simulink model "Speed_Controller_Test_gr2"  (Simulink 7.0)
settings: Solver=ode4  SolverMode=SingleTasking  StartTime=0.0  StopTime=252  FixedStep=0.01  RelTol=1e-3
InitFcn:
  | tempomat_para
StopFcn:
  | clear;
values from neighbouring files (symbols this model uses):
  A = 1.9    [tempomat_para.m]
  a_Fzg_max = 2    [tempomat_para.m]
  a_Fzg_min = -2    [tempomat_para.m]
  cw = 0.32    [tempomat_para.m]
  gang = [1 2 3 4]    [tempomat_para.m]
  gang_vec = [1 2 3 4]    [tempomat_para.m]
  i_anteil = 5    [tempomat_para.m]
  i_d = 3.42    [tempomat_para.m]
  i_g = [3.91 2.17 1.37 1.00]    [tempomat_para.m]
  lambda_gang = [1.3 1.25  1.17  1.05]    [tempomat_para.m]
  m_Fzg = 1400    [tempomat_para.m]
  M_mot_max = [130 149 163 170 168 166 162 158 150 139 123 80]    [tempomat_para.m]
  M_mot_min = [0 -40]    [tempomat_para.m]
  n_mot0 = 1000    [tempomat_para.m]
  n_mot_max = 1000:500:6500    [tempomat_para.m]
  n_mot_min = [1000 6500]    [tempomat_para.m]
  p_anteil = 100    [tempomat_para.m]
  r_dyn = 0.28    [tempomat_para.m]
  rho = 1.202    [tempomat_para.m]
  t_sch = 0.2    [tempomat_para.m]
  TI = [block '/TI']    [PSTI_callback.m]
  v_Fzg_ms0 = 0    [tempomat_para.m]
undefined symbols (not defined in the file or in its folder): Drossel_mat, getdatatypespecs
libraries: simulink x116, fzgbib x3
(part 6 of 10)

== system Speed_Controller_Test_gr2/Test Specification/R2 Speed Control velocity restoration time after simple  acceleration/deceleration/after (6 seconds)  |V_Des-V_Vhcl <= 1.4|/PAS2/Ra delay ==
  In1 : Inport  OutDataType=sfix(16)  OutScaling=2^0
  Data Type Conversion : DataTypeConversion  OutDataType=sfix(16)  OutScaling=2^0
  Delay : Constant  Value=0  OutDataType=sfix(16)  OutScaling=2^0
  Integer Delay : S-Function  FunctionName=sfix_udelay  Parameters=samptime,vinit,NumDelays,1,1,0  mask(Integer Delay){vinit=0.0, samptime=-1, NumDelays=15}
      mask prompts: vinit "Initial condition:"; samptime "Sample time:"; NumDelays "Number of delays:"
      mask help: Delay a signal N sample periods.
      mask init:
      | if isempty(NumDelays)
      |    NumDelays = 1;
      | end
      mask Display: fprintf(' %d\nZ   ',-1*(NumDelays))
  Switch : Switch  Criteria=u2 ~= 0
  Out1 : Outport  OutDataType=sfix(16)  OutScaling=2^0
  wires:
  Switch/1 -> Data Type Conversion/1
  In1/1 -> Switch/3, Integer Delay/1
  Delay/1 -> Switch/2
  Integer Delay/1 -> Switch/1
  Data Type Conversion/1 -> Out1/1

== system Speed_Controller_Test_gr2/Test Specification/R2 Speed Control velocity restoration time after simple  acceleration/deceleration/after (6 seconds)  |V_Des-V_Vhcl <= 1.4|/PAS2/Rp delay ==
  In1 : Inport  OutDataType=sfix(16)  OutScaling=2^0
  Data Type Conversion : DataTypeConversion  OutDataType=sfix(16)  OutScaling=2^0
  Delay : Constant  Value=600  OutDataType=sfix(16)  OutScaling=2^0
  Integer Delay : S-Function  FunctionName=sfix_udelay  Parameters=samptime,vinit,NumDelays,1,1,0  mask(Integer Delay){vinit=0.0, samptime=-1, NumDelays=600}
      mask prompts: vinit "Initial condition:"; samptime "Sample time:"; NumDelays "Number of delays:"
      mask help: Delay a signal N sample periods.
      mask init:
      | if isempty(NumDelays)
      |    NumDelays = 1;
      | end
      mask Display: fprintf(' %d\nZ   ',-1*(NumDelays))
  Switch : Switch  Criteria=u2 ~= 0
  Out1 : Outport  OutDataType=sfix(16)  OutScaling=2^0
  wires:
  Switch/1 -> Data Type Conversion/1
  In1/1 -> Switch/3, Integer Delay/1
  Delay/1 -> Switch/2
  Integer Delay/1 -> Switch/1
  Data Type Conversion/1 -> Out1/1

== system Speed_Controller_Test_gr2/Test Specification/R2 Speed Control velocity restoration time after simple  acceleration/deceleration/after (6 seconds)  |V_Des-V_Vhcl <= 1.4|/PAS2/Ta delay ==
  In1 : Inport  OutDataType=sfix(16)  OutScaling=2^0
  Data Type Conversion : DataTypeConversion  OutDataType=sfix(16)  OutScaling=2^0
  Delay : Constant  Value=0  OutDataType=sfix(16)  OutScaling=2^0
  Integer Delay : S-Function  FunctionName=sfix_udelay  Parameters=samptime,vinit,NumDelays,1,1,0  mask(Integer Delay){vinit=0.0, samptime=-1, NumDelays=15}
      mask prompts: vinit "Initial condition:"; samptime "Sample time:"; NumDelays "Number of delays:"
      mask help: Delay a signal N sample periods.
      mask init:
      | if isempty(NumDelays)
      |    NumDelays = 1;
      | end
      mask Display: fprintf(' %d\nZ   ',-1*(NumDelays))
  Switch : Switch  Criteria=u2 ~= 0
  Out1 : Outport  OutDataType=sfix(16)  OutScaling=2^0
  wires:
  Switch/1 -> Data Type Conversion/1
  In1/1 -> Switch/3, Integer Delay/1
  Delay/1 -> Switch/2
  Integer Delay/1 -> Switch/1
  Data Type Conversion/1 -> Out1/1

== system Speed_Controller_Test_gr2/Test Specification/R2 Speed Control velocity restoration time after simple  acceleration/deceleration/after (6 seconds)  |V_Des-V_Vhcl <= 1.4|/PAS2/Tp delay ==
  In1 : Inport  OutDataType=sfix(16)  OutScaling=2^0
  Data Type Conversion : DataTypeConversion  OutDataType=sfix(16)  OutScaling=2^0
  Delay : Constant  Value=600  OutDataType=sfix(16)  OutScaling=2^0
  Integer Delay : S-Function  FunctionName=sfix_udelay  Parameters=samptime,vinit,NumDelays,1,1,0  mask(Integer Delay){vinit=0.0, samptime=-1, NumDelays=600}
      mask prompts: vinit "Initial condition:"; samptime "Sample time:"; NumDelays "Number of delays:"
      mask help: Delay a signal N sample periods.
      mask init:
      | if isempty(NumDelays)
      |    NumDelays = 1;
      | end
      mask Display: fprintf(' %d\nZ   ',-1*(NumDelays))
  Switch : Switch  Criteria=u2 ~= 0
  Out1 : Outport  OutDataType=sfix(16)  OutScaling=2^0
  wires:
  Switch/1 -> Data Type Conversion/1
  In1/1 -> Switch/3, Integer Delay/1
  Delay/1 -> Switch/2
  Integer Delay/1 -> Switch/1
  Data Type Conversion/1 -> Out1/1

== system Speed_Controller_Test_gr2/Test Specification/R2 Speed Control velocity restoration time after simple  acceleration/deceleration/after (6 seconds)  |V_Des-V_Vhcl <= 1.4|/PAS2/V delay ==
  In1 : Inport  OutDataType=sfix(16)  OutScaling=2^0
  Data Type Conversion : DataTypeConversion  OutDataType=sfix(16)  OutScaling=2^0
  Delay : Constant  Value=0  OutDataType=sfix(16)  OutScaling=2^0
  Integer Delay : S-Function  FunctionName=sfix_udelay  Parameters=samptime,vinit,NumDelays,1,1,0  mask(Integer Delay){vinit=0.0, samptime=-1, NumDelays=15}
      mask prompts: vinit "Initial condition:"; samptime "Sample time:"; NumDelays "Number of delays:"
      mask help: Delay a signal N sample periods.
      mask init:
      | if isempty(NumDelays)
      |    NumDelays = 1;
      | end
      mask Display: fprintf(' %d\nZ   ',-1*(NumDelays))
  Switch : Switch  Criteria=u2 ~= 0
  Out1 : Outport  OutDataType=sfix(16)  OutScaling=2^0
  wires:
  Switch/1 -> Data Type Conversion/1
  In1/1 -> Switch/3, Integer Delay/1
  Delay/1 -> Switch/2
  Integer Delay/1 -> Switch/1
  Data Type Conversion/1 -> Out1/1

== system Speed_Controller_Test_gr2/Test Specification/R2 Speed Control velocity restoration time after simple  acceleration/deceleration/after (6 seconds)  |V_Des-V_Vhcl <= 1.4|/PAS2/error ==
  Rp : Inport  OutDataType=sfix(16)  OutScaling=2^0
  Tp : Inport  Port=2  OutDataType=sfix(16)  OutScaling=2^0
  A : Inport  Port=3  OutDataType=sfix(16)  OutScaling=2^0
  Ra : Inport  Port=4  OutDataType=sfix(16)  OutScaling=2^0
  Ta : Inport  Port=5  OutDataType=sfix(16)  OutScaling=2^0
  V : Inport  Port=6  OutDataType=sfix(16)  OutScaling=2^0
  Compare To Constant{,2,4,6,8,10} (6 alike) : simulink/Logic and Bit Operations/Compare To Constant  SystemSampleTime=-1  relop===  const=0  LogicOutDataTypeMode=uint8  ZeroCross=off
  Compare To Constant{1,3,5,7,9,11} (6 alike) : simulink/Logic and Bit Operations/Compare To Constant  SystemSampleTime=-1  relop===  const=1  LogicOutDataTypeMode=uint8  ZeroCross=off
  Logical Operator{,1,3..6} (6 alike) : Logic  Operator=NOR  AllPortsSameDT=off  OutDataTypeMode=boolean
  Logical Operator2 : Logic  Operator=OR  Inputs=6  AllPortsSameDT=off  OutDataTypeMode=boolean
  Verror : Outport  OutDataType=sfix(16)  OutScaling=2^0
  wires:
  Compare To Constant9/1 -> Logical Operator5/2
  Compare To Constant8/1 -> Logical Operator5/1
  Ta/1 -> Compare To Constant8/1, Compare To Constant9/1
  Compare To Constant7/1 -> Logical Operator4/2
  Compare To Constant6/1 -> Logical Operator4/1
  Ra/1 -> Compare To Constant7/1, Compare To Constant6/1
  Tp/1 -> Compare To Constant3/1, Compare To Constant2/1
  Rp/1 -> Compare To Constant1/1, Compare To Constant/1
  Logical Operator2/1 -> Verror/1
  Compare To Constant3/1 -> Logical Operator1/2
  Compare To Constant2/1 -> Logical Operator1/1
  Compare To Constant1/1 -> Logical Operator/2
  Compare To Constant/1 -> Logical Operator/1
  Compare To Constant5/1 -> Logical Operator3/2
  Compare To Constant4/1 -> Logical Operator3/1
  A/1 -> Compare To Constant4/1, Compare To Constant5/1
  Compare To Constant11/1 -> Logical Operator6/2
  Compare To Constant10/1 -> Logical Operator6/1
  V/1 -> Compare To Constant10/1, Compare To Constant11/1
  Logical Operator/1 -> Logical Operator2/1
  Logical Operator1/1 -> Logical Operator2/2
  Logical Operator3/1 -> Logical Operator2/3
  Logical Operator4/1 -> Logical Operator2/4
  Logical Operator5/1 -> Logical Operator2/5
  Logical Operator6/1 -> Logical Operator2/6

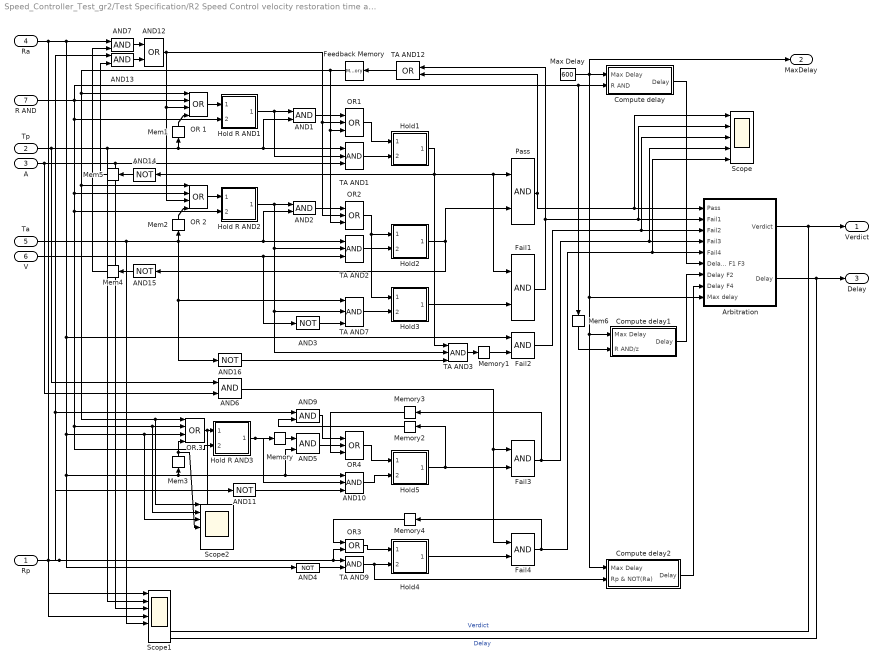
== system Speed_Controller_Test_gr2/Test Specification/R2 Speed Control velocity restoration time after simple  acceleration/deceleration/after (6 seconds)  |V_Des-V_Vhcl <= 1.4|/PAS2/none - pass - fail ==
  Rp : Inport  OutDataType=sfix(16)  OutScaling=2^0
  Tp : Inport  Port=2  OutDataType=sfix(16)  OutScaling=2^0
  A : Inport  Port=3  OutDataType=sfix(16)  OutScaling=2^0
  Ra : Inport  Port=4  OutDataType=sfix(16)  OutScaling=2^0
  Ta : Inport  Port=5  OutDataType=sfix(16)  OutScaling=2^0
  V : Inport  Port=6  OutDataType=sfix(16)  OutScaling=2^0
  R AND : Inport  Port=7  OutDataType=sfix(16)  OutScaling=2^0
  AND{1..2,5..7,9,13} (7 alike) : Logic  AllPortsSameDT=off  OutDataTypeMode=boolean
  AND10 : Logic  Inputs=3  AllPortsSameDT=off  OutDataTypeMode=boolean
  AND{3..4,11,16} (4 alike) : Logic  Operator=NOT  AllPortsSameDT=off  OutDataTypeMode=boolean
  AND12 : Logic  Operator=OR  AllPortsSameDT=off  OutDataTypeMode=boolean
  AND14 : Logic  Orientation=left  Operator=NOT  AllPortsSameDT=off  OutDataTypeMode=boolean
  AND15 : Logic  Orientation=left  Operator=NOT  AllPortsSameDT=off  OutDataTypeMode=boolean
  Arbitration : Subsystem
  Compute delay : Subsystem
  Compute delay1 : Subsystem
  Compute delay2 : Subsystem
  Fail{1..4} (4 alike) : Logic  AllPortsSameDT=off  OutDataTypeMode=boolean
  Feedback Memory : Memory  Orientation=left
  Hold R AND1 : Subsystem  TreatAsAtomicUnit=on
      mask Display: patch(-0.31+[0.4 0.46 0.46 0.54 0.54 0.6 0.6 0.55 0.55 0.45 0.45 0.4],-0.19+[0.85 0.85 0.95 0.95 0.85 0.85 0.87 0.87 0.96 0.96 0.87 0.87],[0 0 0]);
  Hold R AND2 : Subsystem  TreatAsAtomicUnit=on
      mask Display: patch(-0.31+[0.4 0.46 0.46 0.54 0.54 0.6 0.6 0.55 0.55 0.45 0.45 0.4],-0.19+[0.85 0.85 0.95 0.95 0.85 0.85 0.87 0.87 0.96 0.96 0.87 0.87],[0 0 0]);
  Hold R AND3 : Subsystem  TreatAsAtomicUnit=on
      mask Display: patch(-0.31+[0.4 0.46 0.46 0.54 0.54 0.6 0.6 0.55 0.55 0.45 0.45 0.4],-0.19+[0.85 0.85 0.95 0.95 0.85 0.85 0.87 0.87 0.96 0.96 0.87 0.87],[0 0 0]);
  Hold1 : Subsystem  TreatAsAtomicUnit=on
      mask Display: patch(-0.31+[0.4 0.46 0.46 0.54 0.54 0.6 0.6 0.55 0.55 0.45 0.45 0.4],-0.19+[0.85 0.85 0.95 0.95 0.85 0.85 0.87 0.87 0.96 0.96 0.87 0.87],[0 0 0]);
  Hold2 : Subsystem  TreatAsAtomicUnit=on
      mask Display: patch(-0.31+[0.4 0.46 0.46 0.54 0.54 0.6 0.6 0.55 0.55 0.45 0.45 0.4],-0.19+[0.85 0.85 0.95 0.95 0.85 0.85 0.87 0.87 0.96 0.96 0.87 0.87],[0 0 0]);
  Hold3 : Subsystem  TreatAsAtomicUnit=on
      mask Display: patch(-0.31+[0.4 0.46 0.46 0.54 0.54 0.6 0.6 0.55 0.55 0.45 0.45 0.4],-0.19+[0.85 0.85 0.95 0.95 0.85 0.85 0.87 0.87 0.96 0.96 0.87 0.87],[0 0 0]);
  Hold4 : Subsystem  TreatAsAtomicUnit=on
      mask Display: patch(-0.31+[0.4 0.46 0.46 0.54 0.54 0.6 0.6 0.55 0.55 0.45 0.45 0.4],-0.19+[0.85 0.85 0.95 0.95 0.85 0.85 0.87 0.87 0.96 0.96 0.87 0.87],[0 0 0]);
  Hold5 : Subsystem  TreatAsAtomicUnit=on
      mask Display: patch(-0.31+[0.4 0.46 0.46 0.54 0.54 0.6 0.6 0.55 0.55 0.45 0.45 0.4],-0.19+[0.85 0.85 0.95 0.95 0.85 0.85 0.87 0.87 0.96 0.96 0.87 0.87],[0 0 0]);
  Max Delay : Constant  Value=600  OutDataType=sfix(16)  OutScaling=2^0
  Mem1 : Memory  Orientation=up
  Mem2 : Memory  Orientation=up
  Mem3 : Memory  Orientation=up
  Mem4 : Memory  Orientation=left
  Mem5 : Memory  Orientation=left
  Mem6 : Memory  Orientation=down
  Memory : Memory
  Memory1 : Memory
  Memory2 : Memory  Orientation=left
  Memory3 : Memory  Orientation=left
  Memory4 : Memory  Orientation=left
  OR 1 : Logic  Operator=OR  Inputs=4  AllPortsSameDT=off  OutDataTypeMode=boolean
  OR 2 : Logic  Operator=OR  Inputs=4  AllPortsSameDT=off  OutDataTypeMode=boolean
  OR 3 : Logic  Operator=OR  Inputs=4  AllPortsSameDT=off  OutDataTypeMode=boolean
  OR1 : Logic  Operator=OR  Inputs=3  AllPortsSameDT=off  OutDataTypeMode=boolean
  OR2 : Logic  Operator=OR  Inputs=3  AllPortsSameDT=off  OutDataTypeMode=boolean
  OR3 : Logic  Operator=OR  AllPortsSameDT=off  OutDataTypeMode=boolean
  OR4 : Logic  Operator=OR  Inputs=3  AllPortsSameDT=off  OutDataTypeMode=boolean
  Pass : Logic  AllPortsSameDT=off  OutDataTypeMode=boolean
  Scope : Scope  NumInputPorts=5
      settings: YMin=-5~-5~-5~-5~-5  YMax=5~5~5~5~5  SaveName=ScopeData9  MaxDataPoints=1115000
  Scope1 : Scope  NumInputPorts=7
      settings: YMin=-5~-5~-5~-5~-5~-5~-5  YMax=5~5~5~5~5~5~5  SaveName=ScopeData10  MaxDataPoints=1115000
  Scope2 : Scope  NumInputPorts=7
      settings: YMin=-5~-5~-5~-5~-5~-5~-5  YMax=5~5~5~5~5~5~5  SaveName=ScopeData11  MaxDataPoints=1115000
  TA AND{1..3,7} (4 alike) : Logic  Inputs=3  AllPortsSameDT=off  OutDataTypeMode=boolean
  TA AND12 : Logic  Orientation=left  Operator=OR  AllPortsSameDT=off  OutDataTypeMode=boolean
  TA AND9 : Logic  AllPortsSameDT=off  OutDataTypeMode=boolean
  Verdict : Outport  OutDataType=sfix(16)  OutScaling=2^0
  MaxDelay : Outport  Port=2  OutDataType=sfix(16)  OutScaling=2^0
  Delay : Outport  Port=3  OutDataType=sfix(16)  OutScaling=2^0
  wires:
  Arbitration/2(Delay) -> Delay/1, Scope1/7  "Delay"
  Arbitration/1(Verdict) -> Verdict/1, Scope1/6  "Verdict"
  Compute delay2/1(Delay) -> Arbitration/8(Delay F4)
  Compute delay1/1(Delay) -> Arbitration/7(Delay F2)
  Compute delay/1(Delay) -> Arbitration/6(Delay P F1 F3)
  Mem6/1 -> Compute delay1/2(R AND/z)
  AND6/1 -> Fail4/1, Fail3/1
  Max Delay/1 -> MaxDelay/1, Compute delay/1(Max Delay), Arbitration/9(Max delay), Compute delay1/1(Max Delay), Compute delay2/1(Max Delay)
  Memory4/1 -> OR3/1
  OR3/1 -> Hold4/1(" ")
  Pass/1 -> TA AND12/2, Arbitration/1(Pass), Scope/1
  AND16/1 -> TA AND3/3
  Fail1/1 -> TA AND12/1, Arbitration/2(Fail1), Scope/2
  AND15/1 -> Mem4/1
  AND14/1 -> Mem5/1
  Mem5/1 -> AND13/2
  Mem4/1 -> AND7/2
  AND12/1 -> OR2/2, OR1/2, OR 2/3, OR 1/3
  AND13/1 -> AND12/2
  AND7/1 -> AND12/1
  AND5/1 -> OR4/2
  AND10/1 -> Hold5/2("    ")
  AND11/1 -> AND10/3
  Memory3/1 -> OR4/3
  Memory2/1 -> AND9/2
  AND9/1 -> OR4/1
  Memory1/1 -> Fail2/2
  Fail2/1 -> Arbitration/3(Fail2), Scope/3
  Fail4/1 -> Memory4/1, Arbitration/5(Fail4), Scope/5
  Fail3/1 -> Memory3/1, Arbitration/4(Fail3), Scope/4
  TA AND12/1 -> Feedback Memory/1
  Hold5/1("  ") -> Fail3/2, Memory2/1
  Mem3/1 -> OR 3/4, Scope2/4
  OR 3/1 -> Hold R AND3/1(" "), Scope2/5
  Hold R AND3/1("  ") -> Memory/1, AND10/2
  OR4/1 -> Hold5/1(" ")
  Hold4/1("  ") -> Fail4/2
  TA AND9/1 -> Compute delay2/2(Rp & NOT(Ra)), Hold4/2("    ")
  Rp/1 -> OR3/2, TA AND9/1, AND13/1, AND11/1, AND9/1, Scope1/1
  AND4/1 -> TA AND9/2
  Hold3/1("  ") -> Fail1/2
  TA AND3/1 -> Memory1/1
  AND3/1 -> TA AND7/3
  TA AND7/1 -> Hold3/2("    ")
  Mem2/1 -> OR 2/4
  Mem1/1 -> OR 1/4
  Ra/1 -> AND7/1, AND4/1, Mem3/1, AND5/2, AND10/1, OR 3/3, Scope2/3, Fail2/1, Scope1/4
  R AND/1 -> Mem6/1, Compute delay/2(R AND), OR 1/2, Hold R AND1/2("    "), Hold R AND3/2("    "), OR 3/2, Scope2/2, Hold R AND2/2("    "), OR 2/2
  Feedback Memory/1 -> OR2/3, OR1/3, OR 2/1, OR 3/1, Scope2/1, OR 1/1
  AND2/1 -> OR2/1
  Hold R AND2/1("  ") -> TA AND2/2, TA AND7/2, TA AND3/2, AND2/1
  TA AND2/1 -> Hold2/2("    ")
  OR2/1 -> Hold3/1(" "), Hold2/1(" ")
  Hold2/1("  ") -> Pass/2, AND15/1
  V/1 -> TA AND2/3, AND3/1
  OR 2/1 -> Hold R AND2/1(" ")
  Ta/1 -> TA AND2/1, AND2/2, AND16/1, TA AND7/1, Mem2/1, Scope1/5
  AND1/1 -> OR1/1
  Hold R AND1/1("  ") -> TA AND1/2, AND1/1
  TA AND1/1 -> Hold1/2("    ")
  OR1/1 -> Hold1/1(" ")
  Hold1/1("  ") -> TA AND3/1, AND14/1, Fail1/1, Pass/1
  A/1 -> AND6/2, TA AND1/3, Scope1/3
  OR 1/1 -> Hold R AND1/1(" ")
  Tp/1 -> AND6/1, AND1/2, TA AND1/1, Mem1/1, Scope1/2
  Memory/1 -> AND5/1

== system Speed_Controller_Test_gr2/Test Specification/R2 Speed Control velocity restoration time after simple  acceleration/deceleration/after (6 seconds)  |V_Des-V_Vhcl <= 1.4|/R = 2/Active for  6s after R=1  ==
  Signal 2 : Inport  OutDataType=sfix(16)  OutScaling=2^0
  Memory : Memory
  Min Time : Constant  Value=6  OutDataType=sfix(16)  OutScaling=2^0
  Relational Operator2 : RelationalOperator  LogicOutDataTypeMode=boolean
  Scope : Scope  NumInputPorts=5
      settings: YMin=-1~154~-5~80~0  YMax=1~163~5~107.5~110  SaveName=ScopeData13  MaxDataPoints=5000000
  Switch : Switch  Threshold=1
  Time since R = 1 : Subsystem  TreatAsAtomicUnit=on
  Zero : Constant  Value=0  OutDataType=sfix(16)  OutScaling=2^0
  6s after : Outport  OutDataType=sfix(16)  OutScaling=2^0
  wires:
  Relational Operator2/1 -> 6s after/1, Scope/4
  Min Time/1 -> Relational Operator2/1
  Switch/1 -> Relational Operator2/2, Scope/3
  Time since R = 1/1(Trigger) -> Scope/1, Switch/2
  Zero/1 -> Switch/3
  Signal 2/1 -> Time since R = 1/1(Signal)
  Time since R = 1/2(Feature) -> Memory/1
  Memory/1 -> Switch/1, Scope/2

== system Speed_Controller_Test_gr2/Test Specification/R2 Speed Control velocity restoration time after simple  acceleration/deceleration/after (6 seconds)  |V_Des-V_Vhcl <= 1.4|/R = 2/Hold1 ==
  " " : Inport  OutDataType=sfix(16)  OutScaling=2^0
  "    " : Inport  Port=2  OutDataType=sfix(16)  OutScaling=2^0
  Constant : Constant  Value=0  OutDataType=sfix(16)  OutScaling=2^0
  Switch : Switch  Criteria=u2 ~= 0
  "  " : Outport  OutDataType=sfix(16)  OutScaling=2^0
  wires:
  Switch/1 -> "  "/1
  "    "/1 -> Switch/1
  " "/1 -> Switch/2
  Constant/1 -> Switch/3

== system Speed_Controller_Test_gr2/Test Specification/R2 Speed Control velocity restoration time after simple  acceleration/deceleration/after (6 seconds)  |V_Des-V_Vhcl <= 1.4|/R = 2/Hold2 ==
  " " : Inport  OutDataType=sfix(16)  OutScaling=2^0
  "    " : Inport  Port=2  OutDataType=sfix(16)  OutScaling=2^0
  Constant : Constant  Value=0  OutDataType=sfix(16)  OutScaling=2^0
  Switch : Switch  Criteria=u2 ~= 0
  "  " : Outport  OutDataType=sfix(16)  OutScaling=2^0
  wires:
  Switch/1 -> "  "/1
  "    "/1 -> Switch/1
  " "/1 -> Switch/2
  Constant/1 -> Switch/3

== system Speed_Controller_Test_gr2/Test Specification/R2 Speed Control velocity restoration time after simple  acceleration/deceleration/after (6 seconds)  |V_Des-V_Vhcl <= 1.4|/R = 2/R = 1 ==
  In1 : Inport  OutDataType=sfix(16)  OutScaling=2^0
  Bus Selector1 : BusSelector  OutputSignals=R
  Constant : Constant  OutDataType=sfix(16)  OutScaling=2^0
  Relational Operator : RelationalOperator  Operator===  LogicOutDataTypeMode=boolean
  Out1 : Outport  OutDataType=sfix(16)  OutScaling=2^0
  wires:
  In1/1 -> Bus Selector1/1
  Constant/1 -> Relational Operator/2
  Bus Selector1/1 -> Relational Operator/1  "<R>"
  Relational Operator/1 -> Out1/1

== system Speed_Controller_Test_gr2/Test Specification/R1 Speed Control step response/Complete step & CC active + no target & Speed Control active/Complete step detection/Step detection/Active if signals constant for some specified time ==
  Signal1 : Inport  OutDataType=sfix(16)  OutScaling=2^0
  Signal 2 : Inport  Port=2  OutDataType=sfix(16)  OutScaling=2^0
  Logical Operator1 : Logic  AllPortsSameDT=off  OutDataTypeMode=boolean
  Min Time : Constant  Value=10  OutDataType=sfix(16)  OutScaling=2^0
  MinMax : MinMax  Inputs=2  OutDataType=sfix(16)  OutScaling=2^0
  Relational Operator2 : RelationalOperator  Operator=<=  LogicOutDataTypeMode=boolean
  Switch : Switch  Criteria=u2 ~= 0
  Time since signal constant : Subsystem  TreatAsAtomicUnit=on  mask(Feature extraction block){RT=0.001}
      mask prompts: RT "Relative tolerance in %"
      mask help: Detect if the signal value is constant (using the last two signal values) allowing for a user-defined relative deviation
      mask CallbackString:
      | if or( (str2double(get_param(gcb,'RT')) < 0), (str2double(get_param(gcb,'RT')) > 100))
      |     error(['Relative tolerance value (' get_param(gcb,'RT') ') out of range. Please give a value between 0 and 100.']);
      | else
      |     set_param([gcb '/Detect constant/Relative tolerance/Relative Tolerance'],'Value',get_param(gcb,'RT'));
      |     set_param([gcb '/Detect constant'],'RT',get_param(gcb,'RT'));
      | end
  Time since signal constant1 : Subsystem  TreatAsAtomicUnit=on  mask(Feature extraction block){RT=0.001}
      mask prompts: RT "Relative tolerance in %"
      mask help: Detect if the signal value is constant (using the last two signal values) allowing for a user-defined relative deviation
      mask CallbackString:
      | if or( (str2double(get_param(gcb,'RT')) < 0), (str2double(get_param(gcb,'RT')) > 100))
      |     error(['Relative tolerance value (' get_param(gcb,'RT') ') out of range. Please give a value between 0 and 100.']);
      | else
      |     set_param([gcb '/Detect constant/Relative tolerance/Relative Tolerance'],'Value',get_param(gcb,'RT'));
      |     set_param([gcb '/Detect constant'],'RT',get_param(gcb,'RT'));
      | end
  Zero : Constant  Value=0  OutDataType=sfix(16)  OutScaling=2^0
  Constant signals : Outport  OutDataType=sfix(16)  OutScaling=2^0
  wires:
  Zero/1 -> Switch/3
  Logical Operator1/1 -> Switch/2
  MinMax/1 -> Switch/1
  Time since signal constant1/1(Trigger) -> Logical Operator1/2
  Time since signal constant/1(Trigger) -> Logical Operator1/1
  Time since signal constant/2(Feature) -> MinMax/1
  Time since signal constant1/2(Feature) -> MinMax/2
  Switch/1 -> Relational Operator2/2
  Min Time/1 -> Relational Operator2/1
  Relational Operator2/1 -> Constant signals/1
  Signal 2/1 -> Time since signal constant1/1(Signal)
  Signal1/1 -> Time since signal constant/1(Signal)

== system Speed_Controller_Test_gr2/Test Specification/R1 Speed Control step response/Complete step & CC active + no target & Speed Control active/Complete step detection/Step detection/Detect constant ==
  Signal : Inport  OutDataType=sfix(16)  OutScaling=2^0
  Clock : Clock
      settings: Decimation=10
  Constant1 : Constant  Value=0  OutDataTypeMode=boolean  OutDataType=sfix(16)  OutScaling=2^0
  Memory : Memory
  Relative tolerance : Subsystem
  Switch : Switch  Criteria=u2 > Threshold
  Constant : Outport  OutDataType=sfix(16)  OutScaling=2^0
  wires:
  Signal/1 -> Memory/1, Relative tolerance/1(sig)
  Memory/1 -> Relative tolerance/2(ref)
  Constant1/1 -> Switch/3
  Clock/1 -> Switch/2
  Relative tolerance/1(sig == ref) -> Switch/1
  Switch/1 -> Constant/1

== system Speed_Controller_Test_gr2/Test Specification/R1 Speed Control step response/Complete step & CC active + no target & Speed Control active/Complete step detection/Step detection/Detect decrease ==
  Signal : Inport  OutDataType=sfix(16)  OutScaling=2^0
  Clock : Clock
      settings: Decimation=10
  Memory : Memory
  Relational Operator : RelationalOperator  Operator=<  LogicOutDataTypeMode=Specify via dialog
  Switch : Switch  Criteria=u2 > Threshold
  Decrease : Outport  OutDataType=sfix(16)  OutScaling=2^0
  wires:
  Signal/1 -> Relational Operator/1, Memory/1, Switch/3
  Relational Operator/1 -> Decrease/1
  Clock/1 -> Switch/2
  Memory/1 -> Switch/1
  Switch/1 -> Relational Operator/2

== system Speed_Controller_Test_gr2/Test Specification/R1 Speed Control step response/Complete step & CC active + no target & Speed Control active/Complete step detection/Step detection/Detect increase ==
  Signal : Inport  OutDataType=sfix(16)  OutScaling=2^0
  Clock : Clock
      settings: Decimation=10
  Memory : Memory
  Relational Operator : RelationalOperator  Operator=>  LogicOutDataTypeMode=Specify via dialog
  Switch : Switch  Criteria=u2 > Threshold
  Increase : Outport  OutDataType=sfix(16)  OutScaling=2^0
  wires:
  Switch/1 -> Relational Operator/2
  Memory/1 -> Switch/1
  Clock/1 -> Switch/2
  Relational Operator/1 -> Increase/1
  Signal/1 -> Switch/3, Memory/1, Relational Operator/1

== system Speed_Controller_Test_gr2/Test Specification/R1 Speed Control step response/Complete step & CC active + no target & Speed Control active/Complete step detection/Step detection/Detect increase2 ==
  Signal : Inport  OutDataType=sfix(16)  OutScaling=2^0
  Clock : Clock
      settings: Decimation=10
  Memory : Memory
  Relational Operator : RelationalOperator  Operator=>  LogicOutDataTypeMode=Specify via dialog
  Switch : Switch  Criteria=u2 > Threshold
  Increase : Outport  OutDataType=sfix(16)  OutScaling=2^0
  wires:
  Signal/1 -> Relational Operator/1, Memory/1, Switch/3
  Relational Operator/1 -> Increase/1
  Clock/1 -> Switch/2
  Memory/1 -> Switch/1
  Switch/1 -> Relational Operator/2

== system Speed_Controller_Test_gr2/Test Specification/R1 Speed Control step response/Complete step & CC active + no target & Speed Control active/Complete step detection/Step detection/Hold1 ==
  " " : Inport  OutDataType=sfix(16)  OutScaling=2^0
  "    " : Inport  Port=2  OutDataType=sfix(16)  OutScaling=2^0
  Memory : Memory  Orientation=left
  Switch : Switch  Criteria=u2 ~= 0
  "  " : Outport  OutDataType=sfix(16)  OutScaling=2^0
  wires:
  " "/1 -> Switch/2
  "    "/1 -> Switch/1
  Switch/1 -> "  "/1, Memory/1
  Memory/1 -> Switch/3

== system Speed_Controller_Test_gr2/Test Specification/R1 Speed Control step response/Complete step & CC active + no target & Speed Control active/Complete step detection/Step detection reset/Active if signals constant for some specified time ==
  Signal1 : Inport  OutDataType=sfix(16)  OutScaling=2^0
  Signal 2 : Inport  Port=2  OutDataType=sfix(16)  OutScaling=2^0
  Logical Operator1 : Logic  AllPortsSameDT=off  OutDataTypeMode=boolean
  Min Time : Constant  Value=10  OutDataType=sfix(16)  OutScaling=2^0
  MinMax : MinMax  Inputs=2  OutDataType=sfix(16)  OutScaling=2^0
  Relational Operator2 : RelationalOperator  Operator=<=  LogicOutDataTypeMode=boolean
  Switch : Switch  Criteria=u2 ~= 0
  Time since signal constant : Subsystem  TreatAsAtomicUnit=on  mask(Feature extraction block){RT=0.0001}
      mask prompts: RT "Relative tolerance in %"
      mask help: Detect if the signal value is constant (using the last two signal values) allowing for a user-defined relative deviation
      mask CallbackString:
      | if or( (str2double(get_param(gcb,'RT')) < 0), (str2double(get_param(gcb,'RT')) > 100))
      |     error(['Relative tolerance value (' get_param(gcb,'RT') ') out of range. Please give a value between 0 and 100.']);
      | else
      |     set_param([gcb '/Detect constant/Relative tolerance/Relative Tolerance'],'Value',get_param(gcb,'RT'));
      |     set_param([gcb '/Detect constant'],'RT',get_param(gcb,'RT'));
      | end
  Time since signal constant1 : Subsystem  TreatAsAtomicUnit=on  mask(Feature extraction block){RT=0.0001}
      mask prompts: RT "Relative tolerance in %"
      mask help: Detect if the signal value is constant (using the last two signal values) allowing for a user-defined relative deviation
      mask CallbackString:
      | if or( (str2double(get_param(gcb,'RT')) < 0), (str2double(get_param(gcb,'RT')) > 100))
      |     error(['Relative tolerance value (' get_param(gcb,'RT') ') out of range. Please give a value between 0 and 100.']);
      | else
      |     set_param([gcb '/Detect constant/Relative tolerance/Relative Tolerance'],'Value',get_param(gcb,'RT'));
      |     set_param([gcb '/Detect constant'],'RT',get_param(gcb,'RT'));
      | end
  Zero : Constant  Value=0  OutDataType=sfix(16)  OutScaling=2^0
  Constant signals : Outport  OutDataType=sfix(16)  OutScaling=2^0
  wires:
  Signal1/1 -> Time since signal constant/1(Signal)
  Signal 2/1 -> Time since signal constant1/1(Signal)
  Relational Operator2/1 -> Constant signals/1
  Min Time/1 -> Relational Operator2/1
  Switch/1 -> Relational Operator2/2
  Time since signal constant1/2(Feature) -> MinMax/2
  Time since signal constant/2(Feature) -> MinMax/1
  Time since signal constant/1(Trigger) -> Logical Operator1/1
  Time since signal constant1/1(Trigger) -> Logical Operator1/2
  MinMax/1 -> Switch/1
  Logical Operator1/1 -> Switch/2
  Zero/1 -> Switch/3

== system Speed_Controller_Test_gr2/Test Specification/R1 Speed Control step response/Complete step & CC active + no target & Speed Control active/Complete step detection/Step detection reset/Step detection ==
  Signal : Inport  OutDataType=sfix(16)  OutScaling=2^0
  Abs : Abs
  Add : Sum  Inputs=+-  OutDataType=sfix(16)  OutScaling=2^-10
  Clock : Clock
      settings: Decimation=10
  Memory : Memory
  Min step size : Constant  Value=10  OutDataType=sfix(16)  OutScaling=2^0
  Relational Operator : RelationalOperator  LogicOutDataTypeMode=boolean
  Switch : Switch  Criteria=u2 > Threshold
  Step : Outport  OutDataType=sfix(16)  OutScaling=2^0
  wires:
  Add/1 -> Abs/1
  Relational Operator/1 -> Step/1
  Min step size/1 -> Relational Operator/2
  Abs/1 -> Relational Operator/1
  Signal/1 -> Memory/1, Switch/3, Add/1
  Clock/1 -> Switch/2
  Memory/1 -> Switch/1
  Switch/1 -> Add/2

== system Speed_Controller_Test_gr2/Test Specification/R1 Speed Control step response/Complete step & CC active + no target & Speed Control active/PS/TI/Delays1 ==
  In1 : Inport  OutDataType=sfix(16)  OutScaling=2^0
  Delay : Constant  Value=0  OutDataType=sfix(16)  OutScaling=2^0
  Integer Delay : S-Function  FunctionName=sfix_udelay  Parameters=samptime,vinit,NumDelays,1,1,0  mask(Integer Delay){vinit=0.0, samptime=-1, NumDelays=15}
      mask prompts: vinit "Initial condition:"; samptime "Sample time:"; NumDelays "Number of delays:"
      mask help: Delay a signal N sample periods.
      mask init:
      | if isempty(NumDelays)
      |    NumDelays = 1;
      | end
      mask Display: fprintf(' %d\nZ   ',-1*(NumDelays))
  Switch : Switch  Criteria=u2 ~= 0
  Out1 : Outport  OutDataType=sfix(16)  OutScaling=2^0
  wires:
  Integer Delay/1 -> Switch/1
  Delay/1 -> Switch/2
  In1/1 -> Integer Delay/1, Switch/3
  Switch/1 -> Out1/1

== system Speed_Controller_Test_gr2/Test Specification/R1 Speed Control step response/Complete step & CC active + no target & Speed Control active/PS/TI/Delays2 ==
  In1 : Inport  OutDataType=sfix(16)  OutScaling=2^0
  Delay : Constant  Value=0  OutDataType=sfix(16)  OutScaling=2^0
  Integer Delay : S-Function  FunctionName=sfix_udelay  Parameters=samptime,vinit,NumDelays,1,1,0  mask(Integer Delay){vinit=0.0, samptime=-1, NumDelays=15}
      mask prompts: vinit "Initial condition:"; samptime "Sample time:"; NumDelays "Number of delays:"
      mask help: Delay a signal N sample periods.
      mask init:
      | if isempty(NumDelays)
      |    NumDelays = 1;
      | end
      mask Display: fprintf(' %d\nZ   ',-1*(NumDelays))
  Switch : Switch  Criteria=u2 ~= 0
  Out1 : Outport  OutDataType=sfix(16)  OutScaling=2^0
  wires:
  Integer Delay/1 -> Switch/1
  Delay/1 -> Switch/2
  In1/1 -> Integer Delay/1, Switch/3
  Switch/1 -> Out1/1

== system Speed_Controller_Test_gr2/Test Specification/R1 Speed Control step response/Complete step & CC active + no target & Speed Control active/PS/TID/Hold R AND1 ==
  " " : Inport  OutDataType=sfix(16)  OutScaling=2^0
  "    " : Inport  Port=2  OutDataType=sfix(16)  OutScaling=2^0
  Memory : Memory  Orientation=left
  Switch : Switch  Criteria=u2 ~= 0
  "  " : Outport  OutDataType=sfix(16)  OutScaling=2^0
  wires:
  Memory/1 -> Switch/3
  Switch/1 -> Memory/1, "  "/1
  "    "/1 -> Switch/1
  " "/1 -> Switch/2

== system Speed_Controller_Test_gr2/Test Specification/R1 Speed Control step response/Complete step & CC active + no target & Speed Control active/PS/TID/Hold1 ==
  " " : Inport  OutDataType=sfix(16)  OutScaling=2^0
  "    " : Inport  Port=2  OutDataType=sfix(16)  OutScaling=2^0
  Memory : Memory  Orientation=left
  Switch : Switch  Criteria=u2 ~= 0
  "  " : Outport  OutDataType=sfix(16)  OutScaling=2^0
  wires:
  Memory/1 -> Switch/3
  Switch/1 -> Memory/1, "  "/1
  "    "/1 -> Switch/1
  " "/1 -> Switch/2

== system Speed_Controller_Test_gr2/Test Specification/R1 Speed Control step response/Maximum overshoot < 5 &  Steady state error < 5/PAS/Delay bus signals/AD delay ==
  In1 : Inport  OutDataType=sfix(16)  OutScaling=2^0
  Delay : Constant  Value=0  OutDataType=sfix(16)  OutScaling=2^0
  Integer Delay : S-Function  FunctionName=sfix_udelay  Parameters=samptime,vinit,NumDelays,1,1,0  mask(Integer Delay){vinit=0.0, samptime=-1, NumDelays=15}
      mask prompts: vinit "Initial condition:"; samptime "Sample time:"; NumDelays "Number of delays:"
      mask help: Delay a signal N sample periods.
      mask init:
      | if isempty(NumDelays)
      |    NumDelays = 1;
      | end
      mask Display: fprintf(' %d\nZ   ',-1*(NumDelays))
  Switch : Switch  Criteria=u2 ~= 0
  Out1 : Outport  OutDataType=sfix(16)  OutScaling=2^0
  wires:
  Switch/1 -> Out1/1
  In1/1 -> Switch/3, Integer Delay/1
  Delay/1 -> Switch/2
  Integer Delay/1 -> Switch/1

== system Speed_Controller_Test_gr2/Test Specification/R1 Speed Control step response/Maximum overshoot < 5 &  Steady state error < 5/PAS/Delay bus signals/ELL delay ==
  In1 : Inport  OutDataType=sfix(16)  OutScaling=2^0
  Delay : Constant  Value=0  OutDataType=sfix(16)  OutScaling=2^0
  Integer Delay : S-Function  FunctionName=sfix_udelay  Parameters=samptime,vinit,NumDelays,1,1,0  mask(Integer Delay){vinit=0.0, samptime=-1, NumDelays=15}
      mask prompts: vinit "Initial condition:"; samptime "Sample time:"; NumDelays "Number of delays:"
      mask help: Delay a signal N sample periods.
      mask init:
      | if isempty(NumDelays)
      |    NumDelays = 1;
      | end
      mask Display: fprintf(' %d\nZ   ',-1*(NumDelays))
  Switch : Switch  Criteria=u2 ~= 0
  Out1 : Outport  OutDataType=sfix(16)  OutScaling=2^0
  wires:
  Switch/1 -> Out1/1
  In1/1 -> Switch/3, Integer Delay/1
  Delay/1 -> Switch/2
  Integer Delay/1 -> Switch/1

== system Speed_Controller_Test_gr2/Test Specification/R1 Speed Control step response/Maximum overshoot < 5 &  Steady state error < 5/PAS/Delay bus signals/EUL delay ==
  In1 : Inport  OutDataType=sfix(16)  OutScaling=2^0
  Delay : Constant  Value=0  OutDataType=sfix(16)  OutScaling=2^0
  Integer Delay : S-Function  FunctionName=sfix_udelay  Parameters=samptime,vinit,NumDelays,1,1,0  mask(Integer Delay){vinit=0.0, samptime=-1, NumDelays=15}
      mask prompts: vinit "Initial condition:"; samptime "Sample time:"; NumDelays "Number of delays:"
      mask help: Delay a signal N sample periods.
      mask init:
      | if isempty(NumDelays)
      |    NumDelays = 1;
      | end
      mask Display: fprintf(' %d\nZ   ',-1*(NumDelays))
  Switch : Switch  Criteria=u2 ~= 0
  Out1 : Outport  OutDataType=sfix(16)  OutScaling=2^0
  wires:
  Integer Delay/1 -> Switch/1
  Delay/1 -> Switch/2
  In1/1 -> Integer Delay/1, Switch/3
  Switch/1 -> Out1/1

== system Speed_Controller_Test_gr2/Test Specification/R1 Speed Control step response/Maximum overshoot < 5 &  Steady state error < 5/PAS/none - pass - fail/Arbitration ==
  Pass : Inport  OutDataType=sfix(16)  OutScaling=2^0
  Fail1 : Inport  Port=2  OutDataType=sfix(16)  OutScaling=2^0
  Fail2 : Inport  Port=3  OutDataType=sfix(16)  OutScaling=2^0
  Fail3 : Inport  Port=4  OutDataType=sfix(16)  OutScaling=2^0
  Fail4 : Inport  Port=5  OutDataType=sfix(16)  OutScaling=2^0
  Delay P F1 F3 : Inport  Port=6  OutDataType=sfix(16)  OutScaling=2^0
  Delay F2 : Inport  Port=7  OutDataType=sfix(16)  OutScaling=2^0
  Delay F4 : Inport  Port=8  OutDataType=sfix(16)  OutScaling=2^0
  Max delay : Inport  Port=9  OutDataType=sfix(16)  OutScaling=2^0
  Verdict identification : Subsystem
  Verdict selection : Subsystem
  Verdict : Outport  OutDataType=sfix(16)  OutScaling=2^0
  Delay : Outport  Port=2  OutDataType=sfix(16)  OutScaling=2^0
  wires:
  Verdict selection/2(Delay) -> Delay/1
  Verdict selection/1(Verdict) -> Verdict/1
  Max delay/1 -> Verdict selection/6(Max delay)
  Verdict identification/2(V2) -> Verdict selection/2(V2)
  Verdict identification/1(V1) -> Verdict selection/1(V1)
  Delay F4/1 -> Verdict selection/5(Delay F4)
  Delay F2/1 -> Verdict selection/4(Delay F2)
  Delay P F1 F3/1 -> Verdict selection/3(Delay P F1 F3)
  Fail4/1 -> Verdict identification/5(Fail4)
  Fail3/1 -> Verdict identification/4(Fail3)
  Fail2/1 -> Verdict identification/3(Fail2)
  Fail1/1 -> Verdict identification/2(Fail1)
  Pass/1 -> Verdict identification/1(Pass)

== system Speed_Controller_Test_gr2/Test Specification/R1 Speed Control step response/Maximum overshoot < 5 &  Steady state error < 5/PAS/none - pass - fail/Compute delay ==
  Max Delay : Inport  OutDataType=sfix(16)  OutScaling=2^0
  R AND : Inport  Port=2  OutDataType=sfix(16)  OutScaling=2^0
  Clock : Clock
      settings: Decimation=10
  Clock1 : Clock
      settings: Decimation=10
  Divide : Product  Inputs=/*  OutDataType=sfix(16)  OutScaling=2^-10
  Hold1 : Subsystem  TreatAsAtomicUnit=on
      mask Display: patch(-0.31+[0.4 0.46 0.46 0.54 0.54 0.6 0.6 0.55 0.55 0.45 0.45 0.4],-0.19+[0.85 0.85 0.95 0.95 0.85 0.85 0.87 0.87 0.96 0.96 0.87 0.87],[0 0 0]);
  SimStepSize : Constant  Value=0.01  OutDataType=sfix(16)  OutScaling=2^0
  Subtract : Sum  Inputs=-+  OutDataType=sfix(16)  OutScaling=2^-10
  Subtract1 : Sum  Inputs=+-  OutDataType=sfix(16)  OutScaling=2^-10
  Delay : Outport  OutDataType=sfix(16)  OutScaling=2^0
  wires:
  Divide/1 -> Delay/1
  Max Delay/1 -> Subtract/1
  SimStepSize/1 -> Divide/1
  Clock/1 -> Hold1/2("    ")
  Subtract/1 -> Subtract1/2
  Subtract1/1 -> Divide/2
  Clock1/1 -> Subtract1/1
  Hold1/1("  ") -> Subtract/2
  R AND/1 -> Hold1/1(" ")

== system Speed_Controller_Test_gr2/Test Specification/R1 Speed Control step response/Maximum overshoot < 5 &  Steady state error < 5/PAS/none - pass - fail/Compute delay1 ==
  Max Delay : Inport  OutDataType=sfix(16)  OutScaling=2^0
  R AND/z : Inport  Port=2  OutDataType=sfix(16)  OutScaling=2^0
  Add : Sum  OutDataType=sfix(16)  OutScaling=2^-10
  Clock : Clock
      settings: Decimation=10
  Clock1 : Clock
      settings: Decimation=10
  Divide : Product  Inputs=/*  OutDataType=sfix(16)  OutScaling=2^-10
  Hold1 : Subsystem  TreatAsAtomicUnit=on
      mask Display: patch(-0.31+[0.4 0.46 0.46 0.54 0.54 0.6 0.6 0.55 0.55 0.45 0.45 0.4],-0.19+[0.85 0.85 0.95 0.95 0.85 0.85 0.87 0.87 0.96 0.96 0.87 0.87],[0 0 0]);
  SimStepSize : Constant  Value=0.01  OutDataType=sfix(16)  OutScaling=2^0
  Subtract : Sum  Inputs=-+  OutDataType=sfix(16)  OutScaling=2^-10
  Subtract1 : Sum  Inputs=+-  OutDataType=sfix(16)  OutScaling=2^-10
  Unit : Constant  OutDataType=sfix(16)  OutScaling=2^0
  Delay : Outport  OutDataType=sfix(16)  OutScaling=2^0
  wires:
  Divide/1 -> Add/2
  Unit/1 -> Add/1
  Max Delay/1 -> Subtract/1
  SimStepSize/1 -> Divide/1
  Clock/1 -> Hold1/2("    ")
  Subtract/1 -> Subtract1/2
  Subtract1/1 -> Divide/2
  Clock1/1 -> Subtract1/1
  Hold1/1("  ") -> Subtract/2
  R AND/z/1 -> Hold1/1(" ")
  Add/1 -> Delay/1

== system Speed_Controller_Test_gr2/Test Specification/R1 Speed Control step response/Maximum overshoot < 5 &  Steady state error < 5/PAS/none - pass - fail/Compute delay2 ==
  Max Delay : Inport  OutDataType=sfix(16)  OutScaling=2^0
  Rp & NOT(Ra) : Inport  Port=2  OutDataType=sfix(16)  OutScaling=2^0
  Clock : Clock
      settings: Decimation=10
  Clock1 : Clock
      settings: Decimation=10
  Divide : Product  Inputs=/*  OutDataType=sfix(16)  OutScaling=2^-10
  Hold1 : Subsystem  TreatAsAtomicUnit=on
      mask Display: patch(-0.31+[0.4 0.46 0.46 0.54 0.54 0.6 0.6 0.55 0.55 0.45 0.45 0.4],-0.19+[0.85 0.85 0.95 0.95 0.85 0.85 0.87 0.87 0.96 0.96 0.87 0.87],[0 0 0]);
  SimStepSize : Constant  Value=0.01  OutDataType=sfix(16)  OutScaling=2^0
  Subtract : Sum  Inputs=-+  OutDataType=sfix(16)  OutScaling=2^-10
  Subtract1 : Sum  Inputs=+-  OutDataType=sfix(16)  OutScaling=2^-10
  Delay : Outport  OutDataType=sfix(16)  OutScaling=2^0
  wires:
  Divide/1 -> Delay/1
  Rp & NOT(Ra)/1 -> Hold1/1(" ")
  Hold1/1("  ") -> Subtract/2
  Clock1/1 -> Subtract1/1
  Subtract1/1 -> Divide/2
  Subtract/1 -> Subtract1/2
  Clock/1 -> Hold1/2("    ")
  SimStepSize/1 -> Divide/1
  Max Delay/1 -> Subtract/1

== system Speed_Controller_Test_gr2/Test Specification/R1 Speed Control step response/Maximum overshoot < 5 &  Steady state error < 5/PAS/none - pass - fail/Hold R AND1 ==
  " " : Inport  OutDataType=sfix(16)  OutScaling=2^0
  "    " : Inport  Port=2  OutDataType=sfix(16)  OutScaling=2^0
  Memory : Memory  Orientation=left
  Switch : Switch  Criteria=u2 ~= 0
  "  " : Outport  OutDataType=sfix(16)  OutScaling=2^0
  wires:
  Memory/1 -> Switch/3
  Switch/1 -> Memory/1, "  "/1
  "    "/1 -> Switch/1
  " "/1 -> Switch/2

== system Speed_Controller_Test_gr2/Test Specification/R1 Speed Control step response/Maximum overshoot < 5 &  Steady state error < 5/PAS/none - pass - fail/Hold R AND2 ==
  " " : Inport  OutDataType=sfix(16)  OutScaling=2^0
  "    " : Inport  Port=2  OutDataType=sfix(16)  OutScaling=2^0
  Memory : Memory  Orientation=left
  Switch : Switch  Criteria=u2 ~= 0
  "  " : Outport  OutDataType=sfix(16)  OutScaling=2^0
  wires:
  Memory/1 -> Switch/3
  Switch/1 -> Memory/1, "  "/1
  "    "/1 -> Switch/1
  " "/1 -> Switch/2

== system Speed_Controller_Test_gr2/Test Specification/R1 Speed Control step response/Maximum overshoot < 5 &  Steady state error < 5/PAS/none - pass - fail/Hold R AND3 ==
  " " : Inport  OutDataType=sfix(16)  OutScaling=2^0
  "    " : Inport  Port=2  OutDataType=sfix(16)  OutScaling=2^0
  Memory : Memory  Orientation=left
  Switch : Switch  Criteria=u2 ~= 0
  "  " : Outport  OutDataType=sfix(16)  OutScaling=2^0
  wires:
  " "/1 -> Switch/2
  "    "/1 -> Switch/1
  Switch/1 -> "  "/1, Memory/1
  Memory/1 -> Switch/3

== system Speed_Controller_Test_gr2/Test Specification/R1 Speed Control step response/Maximum overshoot < 5 &  Steady state error < 5/PAS/none - pass - fail/Hold1 ==
  " " : Inport  OutDataType=sfix(16)  OutScaling=2^0
  "    " : Inport  Port=2  OutDataType=sfix(16)  OutScaling=2^0
  Memory : Memory  Orientation=left
  Switch : Switch  Criteria=u2 ~= 0
  "  " : Outport  OutDataType=sfix(16)  OutScaling=2^0
  wires:
  Memory/1 -> Switch/3
  Switch/1 -> Memory/1, "  "/1
  "    "/1 -> Switch/1
  " "/1 -> Switch/2

== system Speed_Controller_Test_gr2/Test Specification/R1 Speed Control step response/Maximum overshoot < 5 &  Steady state error < 5/PAS/none - pass - fail/Hold2 ==
  " " : Inport  OutDataType=sfix(16)  OutScaling=2^0
  "    " : Inport  Port=2  OutDataType=sfix(16)  OutScaling=2^0
  Memory : Memory  Orientation=left
  Switch : Switch  Criteria=u2 ~= 0
  "  " : Outport  OutDataType=sfix(16)  OutScaling=2^0
  wires:
  Memory/1 -> Switch/3
  Switch/1 -> Memory/1, "  "/1
  "    "/1 -> Switch/1
  " "/1 -> Switch/2

== system Speed_Controller_Test_gr2/Test Specification/R1 Speed Control step response/Maximum overshoot < 5 &  Steady state error < 5/PAS/none - pass - fail/Hold3 ==
  " " : Inport  OutDataType=sfix(16)  OutScaling=2^0
  "    " : Inport  Port=2  OutDataType=sfix(16)  OutScaling=2^0
  Memory : Memory  Orientation=left
  Switch : Switch  Criteria=u2 ~= 0
  "  " : Outport  OutDataType=sfix(16)  OutScaling=2^0
  wires:
  " "/1 -> Switch/2
  "    "/1 -> Switch/1
  Switch/1 -> "  "/1, Memory/1
  Memory/1 -> Switch/3

== system Speed_Controller_Test_gr2/Test Specification/R1 Speed Control step response/Maximum overshoot < 5 &  Steady state error < 5/PAS/none - pass - fail/Hold4 ==
  " " : Inport  OutDataType=sfix(16)  OutScaling=2^0
  "    " : Inport  Port=2  OutDataType=sfix(16)  OutScaling=2^0
  Memory : Memory  Orientation=left
  Switch : Switch  Criteria=u2 ~= 0
  "  " : Outport  OutDataType=sfix(16)  OutScaling=2^0
  wires:
  Memory/1 -> Switch/3
  Switch/1 -> Memory/1, "  "/1
  "    "/1 -> Switch/1
  " "/1 -> Switch/2

== system Speed_Controller_Test_gr2/Test Specification/R1 Speed Control step response/Maximum overshoot < 5 &  Steady state error < 5/PAS/none - pass - fail/Hold5 ==
  " " : Inport  OutDataType=sfix(16)  OutScaling=2^0
  "    " : Inport  Port=2  OutDataType=sfix(16)  OutScaling=2^0
  Memory : Memory  Orientation=left
  Switch : Switch  Criteria=u2 ~= 0
  "  " : Outport  OutDataType=sfix(16)  OutScaling=2^0
  wires:
  " "/1 -> Switch/2
  "    "/1 -> Switch/1
  Switch/1 -> "  "/1, Memory/1
  Memory/1 -> Switch/3

== system Speed_Controller_Test_gr2/Test Specification/R1 Speed Control step response/Maximum overshoot < 5 &  Steady state error < 5/PAS1/Delay bus signals/AD delay ==
  In1 : Inport  OutDataType=sfix(16)  OutScaling=2^0
  Delay : Constant  Value=0  OutDataType=sfix(16)  OutScaling=2^0
  Integer Delay : S-Function  FunctionName=sfix_udelay  Parameters=samptime,vinit,NumDelays,1,1,0  mask(Integer Delay){vinit=0.0, samptime=-1, NumDelays=15}
      mask prompts: vinit "Initial condition:"; samptime "Sample time:"; NumDelays "Number of delays:"
      mask help: Delay a signal N sample periods.
      mask init:
      | if isempty(NumDelays)
      |    NumDelays = 1;
      | end
      mask Display: fprintf(' %d\nZ   ',-1*(NumDelays))
  Switch : Switch  Criteria=u2 ~= 0
  Out1 : Outport  OutDataType=sfix(16)  OutScaling=2^0
  wires:
  Integer Delay/1 -> Switch/1
  Delay/1 -> Switch/2
  In1/1 -> Integer Delay/1, Switch/3
  Switch/1 -> Out1/1

== system Speed_Controller_Test_gr2/Test Specification/R1 Speed Control step response/Maximum overshoot < 5 &  Steady state error < 5/PAS1/Delay bus signals/ELL delay ==
  In1 : Inport  OutDataType=sfix(16)  OutScaling=2^0
  Delay : Constant  Value=0  OutDataType=sfix(16)  OutScaling=2^0
  Integer Delay : S-Function  FunctionName=sfix_udelay  Parameters=samptime,vinit,NumDelays,1,1,0  mask(Integer Delay){vinit=0.0, samptime=-1, NumDelays=15}
      mask prompts: vinit "Initial condition:"; samptime "Sample time:"; NumDelays "Number of delays:"
      mask help: Delay a signal N sample periods.
      mask init:
      | if isempty(NumDelays)
      |    NumDelays = 1;
      | end
      mask Display: fprintf(' %d\nZ   ',-1*(NumDelays))
  Switch : Switch  Criteria=u2 ~= 0
  Out1 : Outport  OutDataType=sfix(16)  OutScaling=2^0
  wires:
  Integer Delay/1 -> Switch/1
  Delay/1 -> Switch/2
  In1/1 -> Integer Delay/1, Switch/3
  Switch/1 -> Out1/1

== system Speed_Controller_Test_gr2/Test Specification/R1 Speed Control step response/Maximum overshoot < 5 &  Steady state error < 5/PAS1/Delay bus signals/EUL delay ==
  In1 : Inport  OutDataType=sfix(16)  OutScaling=2^0
  Delay : Constant  Value=0  OutDataType=sfix(16)  OutScaling=2^0
  Integer Delay : S-Function  FunctionName=sfix_udelay  Parameters=samptime,vinit,NumDelays,1,1,0  mask(Integer Delay){vinit=0.0, samptime=-1, NumDelays=15}
      mask prompts: vinit "Initial condition:"; samptime "Sample time:"; NumDelays "Number of delays:"
      mask help: Delay a signal N sample periods.
      mask init:
      | if isempty(NumDelays)
      |    NumDelays = 1;
      | end
      mask Display: fprintf(' %d\nZ   ',-1*(NumDelays))
  Switch : Switch  Criteria=u2 ~= 0
  Out1 : Outport  OutDataType=sfix(16)  OutScaling=2^0
  wires:
  Switch/1 -> Out1/1
  In1/1 -> Switch/3, Integer Delay/1
  Delay/1 -> Switch/2
  Integer Delay/1 -> Switch/1

== system Speed_Controller_Test_gr2/Test Specification/R1 Speed Control step response/Maximum overshoot < 5 &  Steady state error < 5/PAS1/none - pass - fail/Arbitration ==
  Pass : Inport  OutDataType=sfix(16)  OutScaling=2^0
  Fail1 : Inport  Port=2  OutDataType=sfix(16)  OutScaling=2^0
  Fail2 : Inport  Port=3  OutDataType=sfix(16)  OutScaling=2^0
  Fail3 : Inport  Port=4  OutDataType=sfix(16)  OutScaling=2^0
  Fail4 : Inport  Port=5  OutDataType=sfix(16)  OutScaling=2^0
  Delay P F1 F3 : Inport  Port=6  OutDataType=sfix(16)  OutScaling=2^0
  Delay F2 : Inport  Port=7  OutDataType=sfix(16)  OutScaling=2^0
  Delay F4 : Inport  Port=8  OutDataType=sfix(16)  OutScaling=2^0
  Max delay : Inport  Port=9  OutDataType=sfix(16)  OutScaling=2^0
  Verdict identification : Subsystem
  Verdict selection : Subsystem
  Verdict : Outport  OutDataType=sfix(16)  OutScaling=2^0
  Delay : Outport  Port=2  OutDataType=sfix(16)  OutScaling=2^0
  wires:
  Pass/1 -> Verdict identification/1(Pass)
  Fail1/1 -> Verdict identification/2(Fail1)
  Fail2/1 -> Verdict identification/3(Fail2)
  Fail3/1 -> Verdict identification/4(Fail3)
  Fail4/1 -> Verdict identification/5(Fail4)
  Delay P F1 F3/1 -> Verdict selection/3(Delay P F1 F3)
  Delay F2/1 -> Verdict selection/4(Delay F2)
  Delay F4/1 -> Verdict selection/5(Delay F4)
  Verdict identification/1(V1) -> Verdict selection/1(V1)
  Verdict identification/2(V2) -> Verdict selection/2(V2)
  Max delay/1 -> Verdict selection/6(Max delay)
  Verdict selection/1(Verdict) -> Verdict/1
  Verdict selection/2(Delay) -> Delay/1
